simulink model "MATE_2level_DriveOversampling"  (R2024b)
settings: Solver=FixedStepDiscrete  StartTime=0.0  StopTime=1  FixedStep=Ts  MaxStep=10e-6  RelTol=1e-3
PostLoadFcn:
  | Ts=2e-6; Ts_Power=30e-6;
InitFcn:
  | Ts=2e-6; Ts_Power=30e-6;
undefined symbols (not defined in the file): DiscIntNeverNeededParam
libraries: nesl_utility x9, simetranss x8, fl_lib x6, ee_lib x6, batteryecm_lib x2, simulink x1
settings Model: ARTEMISmethode_block_infos=$$__separator__$$  Creator=Kyle
settings SolverCC: AlgebraicLoopSolver=TrustRegion
settings DataIOCC: SaveFormat=Array  SignalLoggingSaveFormat=ModelDataLogs  SaveOutput=off  SignalLogging=off  SaveTime=off  ReturnWorkspaceOutputs=off
settings OptimizationCC: OptimizeBlockIOStorage=off  BufferReuse=off  GlobalBufferReuse=off  ExpressionFolding=off  ExpressionDepthLimit=2147483647  LocalBlockOutputs=off  InitFltsAndDblsToZero=on  LifeSpan=inf
settings DebuggingCC: SaveWithParameterizedLinksMsg=none  UnderspecifiedInitializationDetection=Classic  MergeDetectMultiDrivingBlocksExec=none  SignalResolutionControl=TryResolveAllWithWarning  SolverPrmCheckMsg=warning  MultiTaskDSMMsg=warning  MultiTaskCondExecSysMsg=none  FcnCallInpInsideContextMsg=warning  UnconnectedInputMsg=warning  UnconnectedOutputMsg=warning  UnconnectedLineMsg=warning  AllowSymbolicDim=off  StateNameClashWarn=warning  SFUnexpectedBacktrackingDiag=warning  SFNoUnconditionalDefaultTransitionDiag=warning  SFExecutionAtInitializationDiag=none  ArithmeticOperatorsInVariantConditions=warning
settings HardwareCC: ProdBitPerPointer=32  ProdBitPerSizeT=32  ProdBitPerPtrDiffT=32  ProdLargestAtomicFloat=None  ProdIntDivRoundTo=Undefined  ProdEndianess=Unspecified  ProdWordSize=32  ProdHWDeviceType=32-bit Generic  TargetHWDeviceType=32-bit Generic
settings ModelReferenceCC: EnableRefExpFcnMdlSchedulingChecks=on  PropagateSignalLabelsOutOfModel=off
settings SFSimCC: SimUseLocalCustomCode=off  CustomCodeUndefinedFunction=UseInterfaceOnly
settings RTWCC: RTWUseLocalCustomCode=off  GPUComputeCapability=3.5
settings CodeAppCC: StateflowObjectComments=on
settings GRTTargetCC: TargetFcnLib=ansi_tfl_tmw.mat  TargetLangStandard=C89/C90 (ANSI)  CombineOutputUpdateFcns=off  GRTInterface=on
settings ConfigComp: CovMetricSettings=dw  CovSaveCumulativeToWorkspaceVar=on  CovSaveSingleToWorkspaceVar=on  CovExternalEMLEnable=off
settings SimscapeCC: SimscapeNormalizeSystem=off

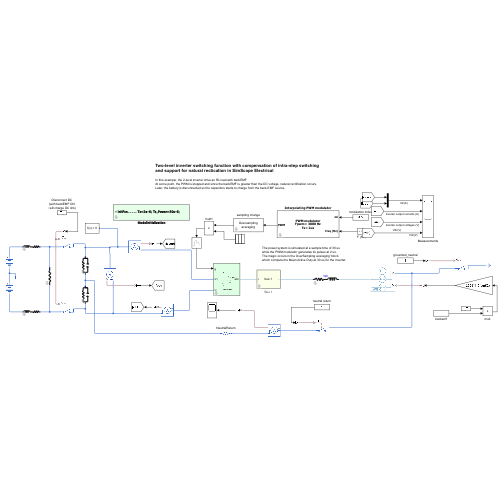
[thumbnail: Simulink's stored preview of the top-level diagram]
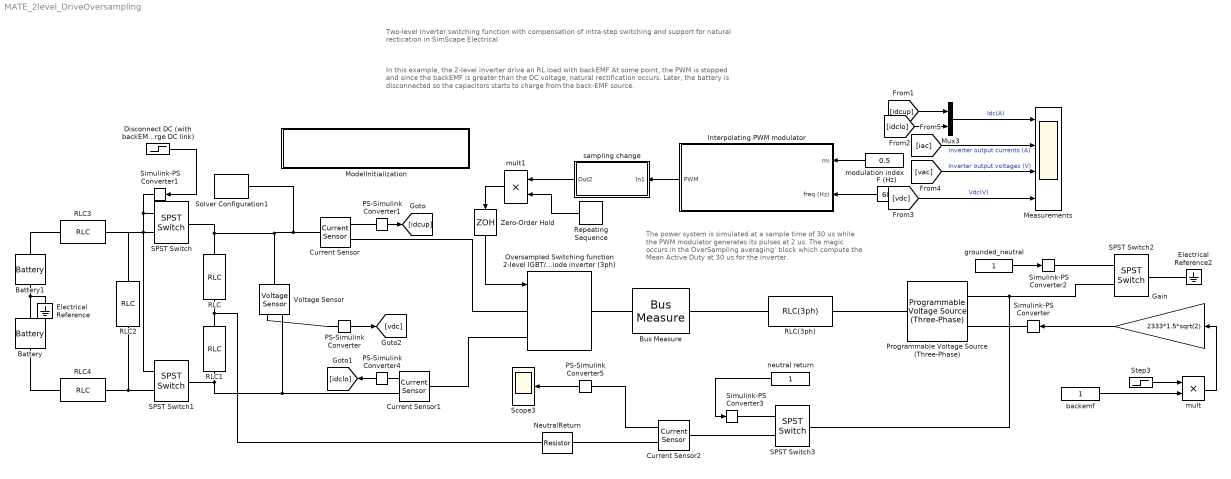
== system MATE_2level_DriveOversampling ==
  note: The power system is simulated at a sample time of 30 us
      | while the PWM modulator generates its pulses at 2 us.
      | The magic occurs in the OverSampling averaging' block
      | which compute the Mean Active Duty at 30 us for the inverter.
  note: In this example, the 2-level inverter drive an RL load with backEMF
      | At some point, the PWM is stopped and since the backEMF is greater than the DC voltage, natural rectification occurs.
      | Later, the battery is disconnected so the capacitors starts to charge from the back-EMF source.
  note: Two-level inverter switching function with compensation of intra-step switching
      | and support for natural rectication in SimScape Electrical
  Battery : batteryecm_lib/Battery  Vnom=2333 V  prm_dir=simscape.enum.battery.prm_dir.disabled  R1_dis=2 Ohm  R1_ch=2 Ohm  R1=0.001 Ohm  prm_AH=simscape.enum.battery.prm_AH.infinite  AH=50 A*hr  V1=11.5 V  AH1=25 A*hr  prm_R2=simscape.enum.battery.prm_R2.disabled  R2=2000 Ohm  Tmeas=298.15 K  charge_measurement_port=simscape.enum.battery.enable.no  prm_dyn=simscape.enum.battery.prm_dyn.off  Rp1=0.005 Ohm  tau1=30 s  Rp2=0.005 Ohm  tau2=30 s  Rp3=0.005 Ohm  tau3=30 s  Rp4=0.005 Ohm  tau4=30 s  Rp5=0.005 Ohm  tau5=30 s  prm_fade=simscape.enum.battery.prm_fade.disabled  N_fade=100  AH_fade=45 A*hr  R1_fade=2.02 Ohm  R1_ch_fade=2.02 Ohm  V1_fade=10.35 V  prm_age=simscape.enum.battery.prm_age.disabled  prm_age_OCV=simscape.enum.battery.prm_age_OCV.OCV  OCV_age=0.9  SOC_age=60  Tmeas_age=298.15 K  delta_time_age_vec=[0] d  temperature_age_vec=[273] K  OCV_scaling_age=2.2134e6  OCV_offset_age=1.632e6  temp_exp_age=0.515833569 V  t_exp_age=0.75  Vnom_T2=12 V  R1_T2=2.2 Ohm  R1_T2_dis=2.2 Ohm  R1_T2_ch=2.2 Ohm  V1_T2=11.4 V  R2_T2=2200 Ohm  Rp1_T2=0.005 Ohm  tau1_T2=30 s  Rp2_T2=0.005 Ohm  tau2_T2=30 s  Rp3_T2=0.005 Ohm  tau3_T2=30 s  Rp4_T2=0.005 Ohm  tau4_T2=30 s  Rp5_T2=0.005 Ohm  tau5_T2=30 s  Tmeas2=273.15 K  thermal_port=simscape.enum.thermaleffects.omit  thermal_mass=30000 J/K  i_specify=off  i_priority=None  i=0 A  i_nominal_specify=off  i_nominal_value=1  i_nominal_unit=A  v_specify=off  v_priority=None  v=0 V  v_nominal_specify=off  v_nominal_value=1  v_nominal_unit=V  charge_specify=off  charge_priority=High  charge=50 A*hr  charge_nominal_specify=off  charge_nominal_value=1  charge_nominal_unit=A*hr  num_cycles_specify=off  num_cycles_priority=High  num_cycles=0  num_cycles_nominal_specify=off  num_cycles_nominal_value=1  num_cycles_nominal_unit=1  temperature_specify=off  temperature_priority=High  temperature=298.15 K  temperature_nominal_specify=off  temperature_nominal_value=1  temperature_nominal_unit=K
  Battery1 : batteryecm_lib/Battery  Vnom=2333 V  prm_dir=simscape.enum.battery.prm_dir.disabled  R1_dis=2 Ohm  R1_ch=2 Ohm  R1=0.001 Ohm  prm_AH=simscape.enum.battery.prm_AH.infinite  AH=50 A*hr  V1=11.5 V  AH1=25 A*hr  prm_R2=simscape.enum.battery.prm_R2.disabled  R2=2000 Ohm  Tmeas=298.15 K  charge_measurement_port=simscape.enum.battery.enable.no  prm_dyn=simscape.enum.battery.prm_dyn.off  Rp1=0.005 Ohm  tau1=30 s  Rp2=0.005 Ohm  tau2=30 s  Rp3=0.005 Ohm  tau3=30 s  Rp4=0.005 Ohm  tau4=30 s  Rp5=0.005 Ohm  tau5=30 s  prm_fade=simscape.enum.battery.prm_fade.disabled  N_fade=100  AH_fade=45 A*hr  R1_fade=2.02 Ohm  R1_ch_fade=2.02 Ohm  V1_fade=10.35 V  prm_age=simscape.enum.battery.prm_age.disabled  prm_age_OCV=simscape.enum.battery.prm_age_OCV.OCV  OCV_age=0.9  SOC_age=60  Tmeas_age=298.15 K  delta_time_age_vec=[0] d  temperature_age_vec=[273] K  OCV_scaling_age=2.2134e6  OCV_offset_age=1.632e6  temp_exp_age=0.515833569 V  t_exp_age=0.75  Vnom_T2=12 V  R1_T2=2.2 Ohm  R1_T2_dis=2.2 Ohm  R1_T2_ch=2.2 Ohm  V1_T2=11.4 V  R2_T2=2200 Ohm  Rp1_T2=0.005 Ohm  tau1_T2=30 s  Rp2_T2=0.005 Ohm  tau2_T2=30 s  Rp3_T2=0.005 Ohm  tau3_T2=30 s  Rp4_T2=0.005 Ohm  tau4_T2=30 s  Rp5_T2=0.005 Ohm  tau5_T2=30 s  Tmeas2=273.15 K  thermal_port=simscape.enum.thermaleffects.omit  thermal_mass=30000 J/K  i_specify=off  i_priority=None  i=0 A  i_nominal_specify=off  i_nominal_value=1  i_nominal_unit=A  v_specify=off  v_priority=None  v=0 V  v_nominal_specify=off  v_nominal_value=1  v_nominal_unit=V  charge_specify=off  charge_priority=High  charge=50 A*hr  charge_nominal_specify=off  charge_nominal_value=1  charge_nominal_unit=A*hr  num_cycles_specify=off  num_cycles_priority=High  num_cycles=0  num_cycles_nominal_specify=off  num_cycles_nominal_value=1  num_cycles_nominal_unit=1  temperature_specify=off  temperature_priority=High  temperature=298.15 K  temperature_nominal_specify=off  temperature_nominal_value=1  temperature_nominal_unit=K
  Bus Measure : simetranss/Measure/Bus Measure  VoltageMeasurement=phase-to-ground  SetLabelV=on  LabelV=vac  Vpu=off  VpuLL=off  CurrentMeasurement=yes  SetLabelI=on  LabelI=iac  Ipu=off  Pbase=100e6  Vbase=500e3  bnumber=1  dis=off
      settings: AttributesFormatString=Bus %<bnumber>
  Current Sensor : fl_lib/Electrical/Electrical Sensors/Current Sensor
  Current Sensor1 : fl_lib/Electrical/Electrical Sensors/Current Sensor
  Current Sensor2 : fl_lib/Electrical/Electrical Sensors/Current Sensor
  "Disconnect DC (with backEMF ON : will charge DC link)" : Step  Time=0.6  Before=1  After=0  SampleTime=0
  Electrical Reference : fl_lib/Electrical/Electrical Elements/Electrical Reference
  Electrical Reference2 : fl_lib/Electrical/Electrical Elements/Electrical Reference
  F (Hz) : Constant  Value=60
  Gain : Gain  Gain=2333*1.5*sqrt(2)
  Interpolating PWM modulator : Subsystem  Tag=RTEcontrol_s38shd7k88  mask(PWM Generator){Fc=3000, Ts=Ts, Freq=60, Phase=0, Tdead=4e-6}
      mask prompts: Fc "Carrier frequency (Hz):"; Ts "Sample time:"; Freq "Frequency of output voltage (Hz)"; Phase "Phase of output voltage (degrees)"; Tdead "Deadtime (s)"
      mask Display: disp(['PWM modulator' 10 'Fpwm= ' num2str(Fc) ' Hz' 10 'Ts= ' num2str(Ts*1e6) 'us'])
  Measurements : Scope  NumInputPorts=4
  ModelInitialization : Subsystem  mask(Model Functions){InitFcnX=Ts=2e-6; Ts_Power=30e-6;, prel=off, posl=on, inif=on, strf=off}
      mask prompts: InitFcnX "Initialisation"; prel "Preload Function"; posl "PostLoad Function"; inif "InitFcn"; strf "StartFcn"
      mask init:
      | if prel==1
      | 	set_param(bdroot, 'PreLoadFcn', InitFcnX);
      | else
      | 	set_param(bdroot, 'PreLoadFcn', '');
      | end
      | if inif==1
      | 	set_param(bdroot, 'InitFcn', InitFcnX);
      | else
      | 	set_param(bdroot, 'InitFcn', '');
      | end
      | if strf==1
      | 	set_param(bdroot, 'StartFcn', InitFcnX);
      | else
      | 	set_param(bdroot, 'StartFcn', '');
      | end
      | if posl==1
      | 	set_param(bdroot, 'PostLoadFcn', InitFcnX);
      | else
      | 	set_param(bdroot, 'PostLoadFcn', '');
      | end
      | PLF = get_param(bdroot, 'PreLoadFcn');
      | IF = get_param(bdroot, 'InitFcn');
      | SF = get_param(bdroot, 'StartFcn');
      | 
      | 
      | pos = get_param(gcb, 'Position');
      | width = pos(3) - pos(1); height = pos(4) - pos(2);
      mask Display:
      | text(5, height*0.5, [ ...
      |   ...
      | '- InitFcn. . . . . '  get_param(bdroot, 'InitFcn')  ...
      | ], ...
      | 'horizontalAlignment', 'left', 'verticalAlignment', 'middle') ;
  Mux3 : Mux  Inputs=2
  NeutralReturn : ee_lib/Passive/Resistor  R=1e-4 Ohm  enable_R_tol=ee.enum.toleranceApplication.none  R_tol=5  tol_distribution=ee.enum.toleranceDistribution.uniform  nSigma=4  enable_operating_limits=ee.enum.enable.no  operating_limit_action=ee.enum.passive.reportOpLim.warn  power_rating=1 W  max_working_voltage=100 V  noise_mode=ee.enum.sources.noise.Disabled  Tdevice=25 degC  sample_time=1e-3 s  repeatability=ee.enum.ic.repeatability.notRepeatable  user_seed=0  auto_seed=415452298  fault_action=simscape.enum.assert.action.none  t_fault=1 s  power_derating_T1=70 degC  power_derating_T2=155 degC  operating_temperature_range_vec=[-50, 150] degC  alpha=3.93e-3 1/K  Tmeas=25 degC  thermal_mass=100 J/K  temperature_specify=off  temperature_priority=High  temperature=298.15 K  temperature_nominal_specify=off  temperature_nominal_value=1  temperature_nominal_unit=K
  Oversampled Switching function 2-level IGBT/diode inverter (3ph) : simetranss/Power converters/Oversampled Switching function 2-level IGBT//diode inverter (3ph)  Ron=1e-3  Rsnubber=100  Csnubber=1e-6  Vf=1  Ts=Ts_Power
  PS-Simulink Converter{,1,4..5} (4 alike) : nesl_utility/PS-Simulink Converter  PhysicalDomain=network_engine_domain  SubClassName=ps_output  LeftPortType=input  RightPortType=output  PseudoPeriodic=off  Frequencies=[]  VectorFormat=inherit  Unit=inherit  AffineConversion=off
  Programmable Voltage Source (Three-Phase) : ee_lib/Sources/Programmable Voltage Source (Three-Phase)  magnitude_type=ee.enum.timechanging.external  vline_rms=100 V  magn_ramp=1 V/s  magn_step=1 V  magn_modu_magn=1 V  magn_modu_freq=1 Hz  magn_t1=1 s  magn_t2=2 s  frequency_type=ee.enum.timechanging.constant  freq=60 Hz  freq_ramp=1 Hz/s  freq_step=1 Hz  freq_modu_magn=1 Hz  freq_modu_freq=1 Hz  freq_t1=1 s  freq_t2=2 s  phase_type=ee.enum.timechanging.constant  shift=0 deg  phase_ramp=1 deg/s  phase_step=1 deg  phase_modu_magn=1 deg  phase_modu_freq=1 Hz  phase_t1=1 s  phase_t2=2 s  impedance_option=1  SShortCircuit=1e6 A*V  XR=15  R=0.01 Ohm  L=3.97e-4 H  G_parasitic=1e-6 1/Ohm  harmonic_option=0  harmonic_orders=[5, 7, 11, 13]  harmonic_ratios=[.1, .1, .1, .1]  harmonic_shifts=[0, 0, 0, 0] deg  harmonic_sequences=[1, 1, 1, 1]  harmonic_t1=-inf s  harmonic_t2=inf s  I_specify=off  I_priority=None  I=[0, 0, 0] A  I_nominal_specify=off  I_nominal_value=1  I_nominal_unit=A  V_specify=off  V_priority=None  V=[0, 0, 0] V  V_nominal_specify=off  V_nominal_value=1  V_nominal_unit=V
      settings: InternalSimscapePortConfiguration="{\"Bottom\":[],\"Left\":[{\"id\":\"ext_magn\",\"label\":\"M\",\"type\":\"input\"},{\"id\":\"n\",\"label\":\"n\",\"type\":\"foundation.electrical.electrical\"}],\"Right\":[{\"id\":\"N\",\"label\":\"~\",\"type\":\"foundation.electrical.three_phase\"}],\"Top\":[]}"
  RLC : simetranss/Passive/RLC  BranchType=RC  SerPar=Parallel  Resistance=4e3  Inductance=1e-3  Capacitance=10e-3  Ropen=1e9
  RLC(3ph) : simetranss/Passive/RLC(3ph)  BranchType=RL  SerPar=Series  Resistance=5  Inductance=10e-3  Capacitance=1e-6  Ropen=1e9
  RLC1 : simetranss/Passive/RLC  BranchType=RC  SerPar=Parallel  Resistance=4e3  Inductance=1e-3  Capacitance=10e-3  Ropen=1e9
  RLC2 : simetranss/Passive/RLC  BranchType=R  SerPar=Parallel  Resistance=50e3  Inductance=1e-3  Capacitance=10e-3  Ropen=1e9
  RLC3 : simetranss/Passive/RLC  BranchType=RL  SerPar=Series  Resistance=0.003  Inductance=1e-4  Capacitance=10e-3  Ropen=1e9
  RLC4 : simetranss/Passive/RLC  BranchType=RL  SerPar=Series  Resistance=0.003  Inductance=1e-4  Capacitance=10e-3  Ropen=1e9
  Repeating Sequence : simulink/Sources/Repeating Sequence  rep_seq_t="[0 0.1 0.1+Ts  0.4 0.4+Ts 10]"  rep_seq_y="[0  0  1            1     0       0]"
  SPST Switch : ee_lib/Switches & Breakers/SPST Switch  R_closed=1e-3 Ohm  G_open=1e-6 S  Threshold=0.5 V  Width=0 V  model_dynamics=0  t_on=1e-3 s  t_off=1e-3 s  initial_vT=0 V
      settings: InternalSimscapePortConfiguration="{\"Bottom\":[],\"Left\":[{\"id\":\"vT\",\"label\":\"vT\",\"type\":\"input\"},{\"id\":\"p\",\"label\":\"\",\"type\":\"foundation.electrical.electrical\"}],\"Right\":[{\"id\":\"n\",\"label\":\"\",\"type\":\"foundation.electrical.electrical\"}],\"Top\":[]}"
  SPST Switch1 : ee_lib/Switches & Breakers/SPST Switch  R_closed=1e-3 Ohm  G_open=1e-6 S  Threshold=0.5 V  Width=0 V  model_dynamics=0  t_on=1e-3 s  t_off=1e-3 s  initial_vT=0 V
      settings: InternalSimscapePortConfiguration="{\"Bottom\":[],\"Left\":[{\"id\":\"vT\",\"label\":\"vT\",\"type\":\"input\"},{\"id\":\"p\",\"label\":\"\",\"type\":\"foundation.electrical.electrical\"}],\"Right\":[{\"id\":\"n\",\"label\":\"\",\"type\":\"foundation.electrical.electrical\"}],\"Top\":[]}"
  SPST Switch2 : ee_lib/Switches & Breakers/SPST Switch  R_closed=1e-3 Ohm  G_open=1e-4 S  Threshold=0.5 V  Width=0 V  model_dynamics=0  t_on=1e-3 s  t_off=1e-3 s  initial_vT=0 V
      settings: InternalSimscapePortConfiguration="{\"Bottom\":[],\"Left\":[{\"id\":\"vT\",\"label\":\"vT\",\"type\":\"input\"},{\"id\":\"p\",\"label\":\"\",\"type\":\"foundation.electrical.electrical\"}],\"Right\":[{\"id\":\"n\",\"label\":\"\",\"type\":\"foundation.electrical.electrical\"}],\"Top\":[]}"
  SPST Switch3 : ee_lib/Switches & Breakers/SPST Switch  R_closed=1e-3 Ohm  G_open=1e-6 S  Threshold=0.5 V  Width=0 V  model_dynamics=0  t_on=1e-3 s  t_off=1e-3 s  initial_vT=0 V
      settings: InternalSimscapePortConfiguration="{\"Bottom\":[],\"Left\":[{\"id\":\"vT\",\"label\":\"vT\",\"type\":\"input\"},{\"id\":\"p\",\"label\":\"\",\"type\":\"foundation.electrical.electrical\"}],\"Right\":[{\"id\":\"n\",\"label\":\"\",\"type\":\"foundation.electrical.electrical\"}],\"Top\":[]}"
  Scope3 : Scope
  Simulink-PS Converter{,1..3} (4 alike) : nesl_utility/Simulink-PS Converter  PhysicalDomain=network_engine_domain  SubClassName=ps_input  LeftPortType=input  RightPortType=output  PseudoPeriodic=off  Frequencies=[]  NoiseDistribution=none  NoiseParameters=[]  Unit=1  AffineConversion=off  FilteringAndDerivatives=provide  SimscapeFilterOrder=1  InputFilterTimeConstant=0.001  UdotUserProvided=0
  Solver Configuration1 : nesl_utility/Solver Configuration  PhysicalDomain=network_engine_domain  SubClassName=solver  LeftPortType=input  RightPortType=generic  Tones=[]  Harmonics=[]  SimulateNoise=off  Profile=off  UseLocalSampling=off  EnableSwitchedLinearOptims=on  FrequencyDomain=off  UseCCode=off  RelTol=0.001  AbsTol=1e-06  MinStep=1e-09  ToWorkspace=off  RevertToSquareIcSolve=off  NumHomotopyIterations=100  PhasorMode=off  PhasorModeNumHarmonics=1  ConsistencySolver=NEWTON_FTOL  IndexReductionMethod=DerivativeReplacement  DoDC=off  ResidualTolerance=0.001  ConsistencyTolSource=GLOBAL  ConsistencyAbsTol=0.001  ConsistencyRelTol=0.001  ConsistencyTolFactor=0.001  UseLocalSolver=on  LocalSolverChoice=NE_PARTITIONING_ADVANCER  ResolveIndetEquations=off  FunctionEvalNumThread=1  LocalSolverSampleTime=Ts_Power  DoFixedCost=on  MaxNonlinIter=1  MaxModeIter=2  ComputeImpulses=off  ImpulseIterations=2  LinearAlgebra=Sparse  LinearAlgebraNumThread=0  EquationFormulation=NE_TIME_EF  DelaysMemoryBudget=1024  AutomaticFiltering=off  FilteringTimeConstant=0.001  PartitionStorageMethod=AS_NEEDED  PartitionMemoryBudget=1024  PartitionMethod=ROBUST  MultibodyUseLocalSolver=off  MultibodyLocalSolverChoice=ODE1  MultibodyLocalSolverSampleTime=0.001
  Step3 : Step  Time=0.08  SampleTime=0
  Voltage Sensor : fl_lib/Electrical/Electrical Sensors/Voltage Sensor
  Zero-Order Hold : ZeroOrderHold  SampleTime=Ts_Power
  backemf : Constant
  grounded_neutral : Constant
  modulation index : Constant  Value=0.5
  mult : Product
  mult1 : Product
  neutral return : Constant
  sampling change : Subsystem  mask(Oversampling converter){rat=15, Ts=Ts}
      mask prompts: rat "Slower time step ratio"; Ts "Sample time (s)"
      mask TypeOptions rat: 2 | 3 | 4 | 5 | 10 | 15
      mask Display: disp(['Oversampling' 10 'averaging'])
  wires:
  "Disconnect DC (with backEMF ON : will charge DC link)"/1 -> Simulink-PS Converter1/1
  Gain/1 -> Simulink-PS Converter/1
  F (Hz)/1 -> Interpolating PWM modulator/2(freq (Hz))
  modulation index/1 -> Interpolating PWM modulator/1(mi)
  mult1/1 -> Zero-Order Hold/1
  Repeating Sequence/1 -> mult1/2
  neutral return/1 -> Simulink-PS Converter3/1
  backemf/1 -> mult/2
  mult/1 -> Gain/1
  Step3/1 -> mult/1
  [vdc] -> Measurements/4  "Vdc(V)"
  grounded_neutral/1 -> Simulink-PS Converter2/1
  Mux3/1 -> Measurements/1  "Idc(A)"
  PS-Simulink Converter5/1 -> Scope3/1
  PS-Simulink Converter1/1 -> [idcup]
  PS-Simulink Converter4/1 -> [idclo]
  PS-Simulink Converter/1 -> [vdc]
  [idcup] -> Mux3/1
  [idclo] -> Mux3/2
  [iac] -> Measurements/2  "Inverter output currents (A)"
  [vac] -> Measurements/3  "Inverter output voltages (V)"
  Interpolating PWM modulator/1(PWM) -> sampling change/1(In1)
  Zero-Order Hold/1 -> Oversampled Switching function 2-level IGBT/diode inverter (3ph)/1
  sampling change/1(Out2) -> mult1/1
  connections:
  Simulink-PS Converter1/RConn1 -- SPST Switch1/LConn1 -- SPST Switch/LConn1
  Current Sensor1/RConn1 -- PS-Simulink Converter4/LConn1
  Simulink-PS Converter/RConn1 -- Programmable Voltage Source (Three-Phase)/LConn1
  Programmable Voltage Source (Three-Phase)/LConn2 -- SPST Switch2/LConn2 -- SPST Switch3/RConn1
  Oversampled Switching function 2-level IGBT/diode inverter (3ph)/LConn2 -- Current Sensor1/LConn1
  Oversampled Switching function 2-level IGBT/diode inverter (3ph)/LConn1 -- Current Sensor/RConn2
  PS-Simulink Converter1/LConn1 -- Current Sensor/RConn1
  PS-Simulink Converter/LConn1 -- Voltage Sensor/RConn1
  SPST Switch1/RConn1 -- Voltage Sensor/RConn2 -- Current Sensor1/RConn2 -- RLC1/RConn1
  SPST Switch/RConn1 -- RLC/LConn1 -- Voltage Sensor/LConn1 -- Solver Configuration1/RConn1 -- Current Sensor/LConn1
  RLC2/RConn1 -- RLC4/LConn1 -- SPST Switch1/LConn2
  SPST Switch/LConn2 -- RLC2/LConn1 -- RLC3/LConn1
  RLC4/RConn1 -- Battery/RConn1
  RLC3/RConn1 -- Battery1/LConn1
  Battery/LConn1 -- Electrical Reference/LConn1 -- Battery1/RConn1
  RLC/RConn1 -- RLC1/LConn1 -- NeutralReturn/RConn1
  RLC(3ph)/LConn1 -- Bus Measure/RConn1
  RLC(3ph)/RConn1 -- Programmable Voltage Source (Three-Phase)/RConn1
  Bus Measure/LConn1 -- Oversampled Switching function 2-level IGBT/diode inverter (3ph)/RConn1
  SPST Switch2/RConn1 -- Electrical Reference2/LConn1
  Simulink-PS Converter2/RConn1 -- SPST Switch2/LConn1
  Current Sensor2/RConn2 -- NeutralReturn/LConn1
  SPST Switch3/LConn2 -- Current Sensor2/LConn1
  Simulink-PS Converter3/RConn1 -- SPST Switch3/LConn1
  Current Sensor2/RConn1 -- PS-Simulink Converter5/LConn1

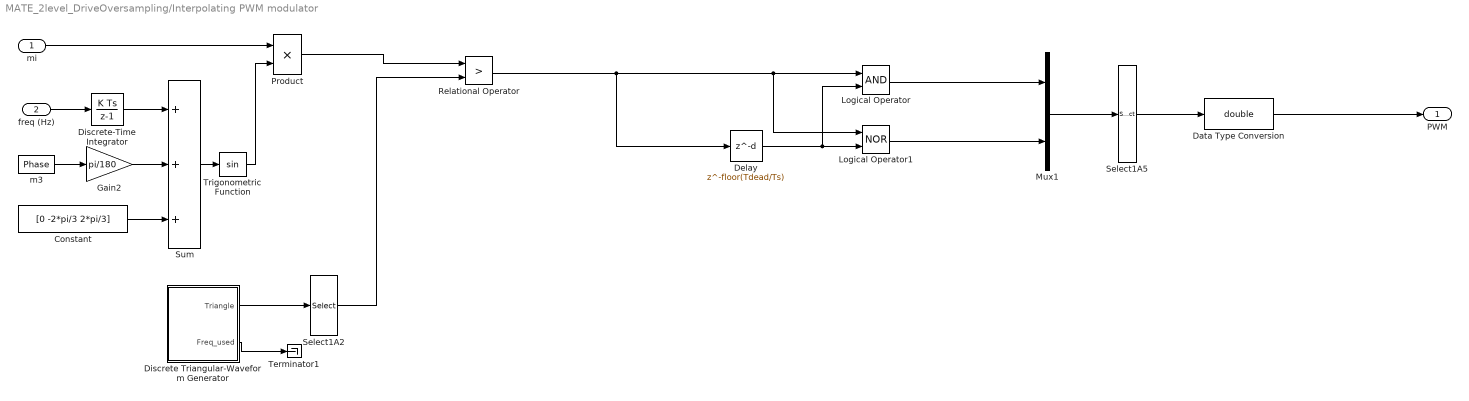
== system MATE_2level_DriveOversampling/Interpolating PWM modulator ==
  mi : Inport  OutDataTypeStr=double
  freq (Hz) : Inport  Port=2  OutDataTypeStr=double
  Constant : Constant  Value=[0 -2*pi/3 2*pi/3]
  Data Type Conversion : DataTypeConversion  OutDataTypeStr=double  SaturateOnIntegerOverflow=off  RndMeth=Floor
  Delay : Delay  DelayLength=floor(Tdead/Ts)  SampleTime=Ts
  Discrete Triangular-Waveform Generator : Subsystem  mask(Discrete Triangular-Waveform  Generator){Freq=Fc, Vpeak=1, Ts=Ts}
      mask prompts: Freq "Frequency (Hz):"; Vpeak "Peak value:"; Ts "Sample time:"
      mask init:
      | NumberStepsRounded=round(1/Freq/Ts);
      | % Selection of an even number of steps
      | if mod(NumberStepsRounded,2)==0
      |    NumberSteps=NumberStepsRounded;
      | else
      |    NumberSteps=NumberStepsRounded+1;
      | end
      | Freq_used=1/(NumberSteps*Ts);
  Discrete-Time Integrator : DiscreteIntegrator  gainval=2*pi  SampleTime=Ts  ICPrevOutput=DiscIntNeverNeededParam  ICPrevScaledInput=DiscIntNeverNeededParam
  Gain2 : Gain  Gain=pi/180  SaturateOnIntegerOverflow=on  OutDataTypeStr=Inherit: Same as input  ParamDataTypeStr=Inherit: Same as input
  Logical Operator : Logic  AllPortsSameDT=off  OutDataTypeStr=boolean
  Logical Operator1 : Logic  Operator=NOR  AllPortsSameDT=off  OutDataTypeStr=boolean
  Mux1 : Mux  Inputs=2
  Product : Product  InputSameDT=on  SaturateOnIntegerOverflow=on  OutDataTypeStr=Inherit: Same as first input
  Relational Operator : RelationalOperator  Operator=>  OutDataTypeStr=boolean  RndMeth=Simplest  InputSameDT=off
  Select1A2 : Selector  InputPortWidth=1  IndexOptions=Index vector (dialog)  Indices=[1 1 1]  OutputSizes=1
  Select1A5 : Selector  InputPortWidth=6  IndexOptions=Index vector (dialog)  Indices=[1 4 2 5 3 6]  OutputSizes=1
  Sum : Sum  Inputs=+++  InputSameDT=on  SaturateOnIntegerOverflow=on  OutDataTypeStr=Inherit: Same as first input
  Terminator1 : Terminator
  Trigonometric Function : Trigonometry
  m3 : Constant  Value=Phase
  PWM : Outport
  wires:
  Select1A2/1 -> Relational Operator/2
  Discrete Triangular-Waveform Generator/1(Triangle) -> Select1A2/1
  Discrete Triangular-Waveform Generator/2(Freq_used) -> Terminator1/1
  Product/1 -> Relational Operator/1
  Trigonometric Function/1 -> Product/2
  Sum/1 -> Trigonometric Function/1
  mi/1 -> Product/1
  Constant/1 -> Sum/3
  m3/1 -> Gain2/1
  Gain2/1 -> Sum/2
  Relational Operator/1 -> Delay/1, Logical Operator1/1, Logical Operator/1
  Logical Operator/1 -> Mux1/1
  Logical Operator1/1 -> Mux1/2
  Mux1/1 -> Select1A5/1
  Select1A5/1 -> Data Type Conversion/1
  freq (Hz)/1 -> Discrete-Time Integrator/1
  Discrete-Time Integrator/1 -> Sum/1
  Delay/1 -> Logical Operator/2, Logical Operator1/2
  Data Type Conversion/1 -> PWM/1

== system MATE_2level_DriveOversampling/ModelInitialization ==

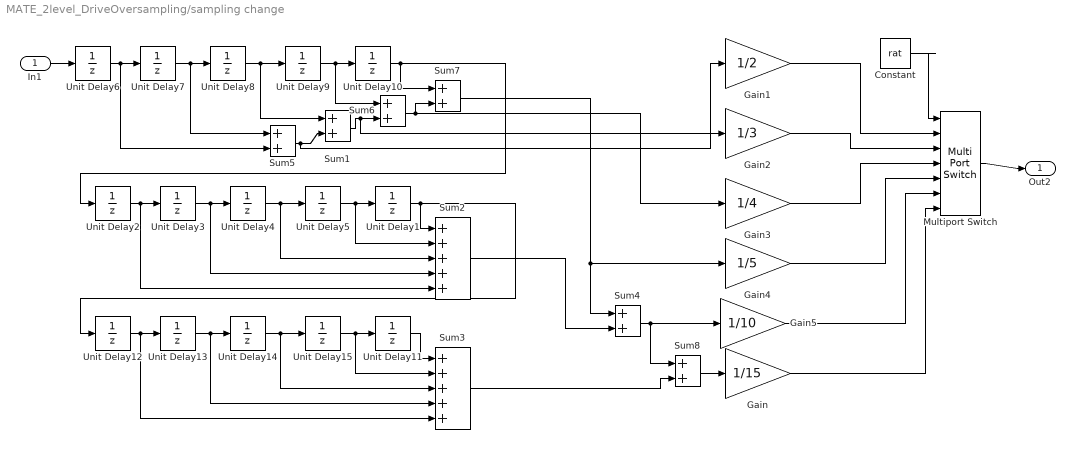
== system MATE_2level_DriveOversampling/sampling change ==
  In1 : Inport
  Constant : Constant  Value=rat
  Gain : Gain  Gain=1/15
  Gain1 : Gain  Gain=1/2
  Gain2 : Gain  Gain=1/3
  Gain3 : Gain  Gain=1/4
  Gain4 : Gain  Gain=1/5
  Gain5 : Gain  Gain=1/10
  Multiport Switch : MultiPortSwitch  Inputs=6  SaturateOnIntegerOverflow=off  InputSameDT=off
  Sum{1,4..8} (6 alike) : Sum  Inputs=2
  Sum2 : Sum  Inputs=5
  Sum3 : Sum  Inputs=5
  Unit Delay{1..15} (15 alike) : UnitDelay  SampleTime=Ts  HasFrameUpgradeWarning=on
  Out2 : Outport
  wires:
  Unit Delay6/1 -> Unit Delay7/1, Sum5/2
  Unit Delay7/1 -> Unit Delay8/1, Sum5/1
  Unit Delay8/1 -> Unit Delay9/1, Sum1/1
  Unit Delay9/1 -> Unit Delay10/1, Sum6/1
  Unit Delay10/1 -> Unit Delay2/1, Sum7/1
  In1/1 -> Unit Delay6/1
  Unit Delay2/1 -> Sum2/5, Unit Delay3/1
  Unit Delay3/1 -> Sum2/4, Unit Delay4/1
  Unit Delay4/1 -> Sum2/3, Unit Delay5/1
  Unit Delay5/1 -> Sum2/2, Unit Delay1/1
  Unit Delay1/1 -> Sum2/1, Unit Delay12/1
  Unit Delay12/1 -> Unit Delay13/1, Sum3/5
  Unit Delay13/1 -> Unit Delay14/1, Sum3/4
  Unit Delay14/1 -> Unit Delay15/1, Sum3/3
  Unit Delay15/1 -> Unit Delay11/1, Sum3/2
  Unit Delay11/1 -> Sum3/1
  Sum2/1 -> Sum4/2
  Sum3/1 -> Sum8/2
  Sum8/1 -> Gain/1
  Sum7/1 -> Gain4/1, Sum4/1
  Sum5/1 -> Sum1/2, Gain1/1
  Sum1/1 -> Sum6/2, Gain2/1
  Sum6/1 -> Sum7/2, Gain3/1
  Sum4/1 -> Gain5/1, Sum8/1
  Gain1/1 -> Multiport Switch/2
  Gain2/1 -> Multiport Switch/3
  Gain3/1 -> Multiport Switch/4
  Gain4/1 -> Multiport Switch/5
  Gain5/1 -> Multiport Switch/6
  Multiport Switch/1 -> Out2/1
  Gain/1 -> Multiport Switch/7
  Constant/1 -> Multiport Switch/1

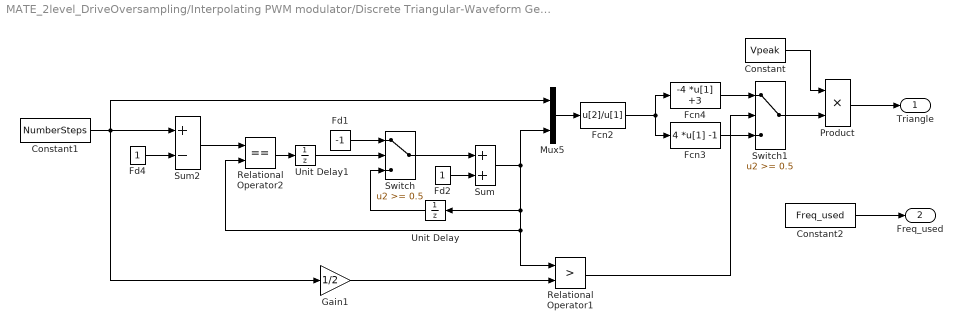
== system MATE_2level_DriveOversampling/Interpolating PWM modulator/Discrete Triangular-Waveform Generator ==
  Constant : Constant  Value=Vpeak
  Constant1 : Constant  Value=NumberSteps
  Constant2 : Constant  Value=Freq_used
  Fcn2 : Fcn  Expr=u[2]/u[1]
  Fcn3 : Fcn  Expr=4 *u[1] -1
  Fcn4 : Fcn  Expr=-4 *u[1] +3
  Fd1 : Constant  Value=-1
  Fd2 : Constant
  Fd4 : Constant
  Gain1 : Gain  Gain=1/2  SaturateOnIntegerOverflow=on  OutDataTypeStr=Inherit: Same as input  ParamDataTypeStr=Inherit: Same as input
  Mux5 : Mux  Inputs=2
  Product : Product  InputSameDT=on  SaturateOnIntegerOverflow=on  OutDataTypeStr=Inherit: Same as first input
  Relational Operator1 : RelationalOperator  Operator=>
  Relational Operator2 : RelationalOperator  Operator===
  Sum : Sum  InputSameDT=on  SaturateOnIntegerOverflow=on  OutDataTypeStr=Inherit: Same as first input
  Sum2 : Sum  Inputs=+-  InputSameDT=on  SaturateOnIntegerOverflow=on  OutDataTypeStr=Inherit: Same as first input
  Switch : Switch  Threshold=0.5
  Switch1 : Switch  Threshold=0.5
  Unit Delay : UnitDelay  SampleTime=Ts  HasFrameUpgradeWarning=on
  Unit Delay1 : UnitDelay  SampleTime=Ts  HasFrameUpgradeWarning=on
  Triangle : Outport  InitialOutput=0
  Freq_used : Outport  Port=2  InitialOutput=0
  wires:
  Product/1 -> Triangle/1
  Switch1/1 -> Product/2
  Constant/1 -> Product/1
  Fd4/1 -> Sum2/2
  Switch/1 -> Sum/1
  Fd2/1 -> Sum/2
  Fd1/1 -> Switch/1
  Unit Delay/1 -> Switch/3
  Unit Delay1/1 -> Switch/2
  Relational Operator2/1 -> Unit Delay1/1
  Sum2/1 -> Relational Operator2/1
  Constant1/1 -> Sum2/1, Mux5/1, Gain1/1
  Sum/1 -> Unit Delay/1, Relational Operator2/2, Relational Operator1/1, Mux5/2
  Fcn2/1 -> Fcn4/1, Fcn3/1
  Mux5/1 -> Fcn2/1
  Fcn4/1 -> Switch1/1
  Fcn3/1 -> Switch1/3
  Gain1/1 -> Relational Operator1/2
  Relational Operator1/1 -> Switch1/2
  Constant2/1 -> Freq_used/1
